simulink model "Question3"  (R2018a)
settings: Solver=VariableStepDiscrete  StartTime=0.0  StopTime=0.5  RelTol=1e-3
libraries: powerlib x17, powerlib_meascontrol x1
settings Model: Creator=bulbu  LastModifiedBy=bulbu

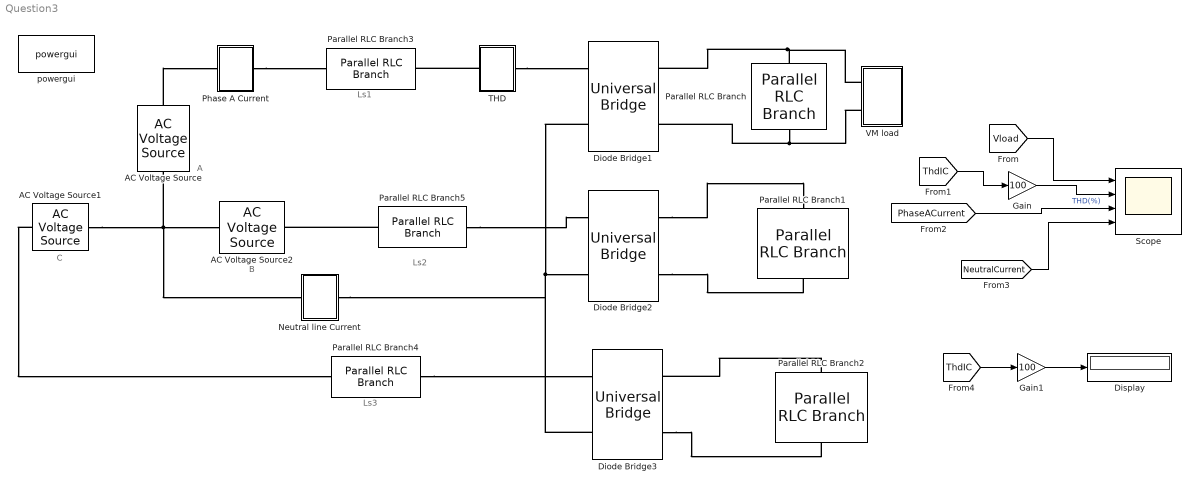
== system Question3 ==
  note: Ls1
  note: C
  note: B
  note: A
  note: Ls2
  note: Ls3
  AC Voltage Source : powerlib/Electrical Sources/AC Voltage Source  Amplitude=326.6  Phase=0  Frequency=50  SampleTime=0  Measurements=None  BusType=swing  Pref=10e3  Qref=0  Qmin=-inf  Qmax=+inf
  AC Voltage Source1 : powerlib/Electrical Sources/AC Voltage Source  Amplitude=326.6  Phase=-120  Frequency=50  SampleTime=0  Measurements=None  BusType=swing  Pref=10e3  Qref=0  Qmin=-inf  Qmax=+inf
  AC Voltage Source2 : powerlib/Electrical Sources/AC Voltage Source  Amplitude=326.6  Phase=120  Frequency=50  SampleTime=0  Measurements=None  BusType=swing  Pref=10e3  Qref=0  Qmin=-inf  Qmax=+inf
  Diode Bridge1 : powerlib/Power Electronics/Universal Bridge  Arms=2  SnubberResistance=1e5  SnubberCapacitance=inf  Device=Diodes  Ron=1e-3  Lon=0  ForwardVoltages="[  0  0  ]"  ForwardVoltage=0  GTOparameters=[ 10e-6 , 20e-6 ]  IGBTparameters=[ 1e-6 , 2e-6 ]  Measurements=None  Measurements_2=None  converterType=Rectifier
  Diode Bridge2 : powerlib/Power Electronics/Universal Bridge  Arms=2  SnubberResistance=1e5  SnubberCapacitance=inf  Device=Diodes  Ron=1e-3  Lon=0  ForwardVoltages="[  0  0  ]"  ForwardVoltage=0  GTOparameters=[ 10e-6 , 20e-6 ]  IGBTparameters=[ 1e-6 , 2e-6 ]  Measurements=None  Measurements_2=None  converterType=Rectifier
  Diode Bridge3 : powerlib/Power Electronics/Universal Bridge  Arms=2  SnubberResistance=1e5  SnubberCapacitance=inf  Device=Diodes  Ron=1e-3  Lon=0  ForwardVoltages="[  0  0  ]"  ForwardVoltage=0  GTOparameters=[ 10e-6 , 20e-6 ]  IGBTparameters=[ 1e-6 , 2e-6 ]  Measurements=None  Measurements_2=None  converterType=Rectifier
  Display : Display
  Gain : Gain  Gain=100
  Gain1 : Gain  Gain=100
  "Neutral line Current " : Subsystem
  Parallel RLC Branch : powerlib/Elements/Parallel RLC Branch  LConnTagsString=a  RConnTagsString=__new0  BranchType=RC  Resistance=200  Inductance=1e-3  SetiL0=off  InitialCurrent=0  Capacitance=470e-6  Setx0=off  InitialVoltage=0  Measurements=None
  Parallel RLC Branch1 : powerlib/Elements/Parallel RLC Branch  LConnTagsString=a  RConnTagsString=__new0  BranchType=RC  Resistance=200  Inductance=1e-3  SetiL0=off  InitialCurrent=0  Capacitance=470e-6  Setx0=off  InitialVoltage=0  Measurements=None
  Parallel RLC Branch2 : powerlib/Elements/Parallel RLC Branch  LConnTagsString=a  RConnTagsString=__new0  BranchType=RC  Resistance=200  Inductance=1e-3  SetiL0=off  InitialCurrent=0  Capacitance=470e-6  Setx0=off  InitialVoltage=0  Measurements=None
  Parallel RLC Branch3 : powerlib/Elements/Parallel RLC Branch  LConnTagsString=a  RConnTagsString=__new0  BranchType=L  Resistance=1  Inductance=600e-6  SetiL0=off  InitialCurrent=0  Capacitance=1e-6  Setx0=off  InitialVoltage=0  Measurements=None
  Parallel RLC Branch4 : powerlib/Elements/Parallel RLC Branch  LConnTagsString=a  RConnTagsString=__new0  BranchType=L  Resistance=1  Inductance=600e-6  SetiL0=off  InitialCurrent=0  Capacitance=1e-6  Setx0=off  InitialVoltage=0  Measurements=None
  Parallel RLC Branch5 : powerlib/Elements/Parallel RLC Branch  LConnTagsString=a  RConnTagsString=__new0  BranchType=L  Resistance=1  Inductance=600e-6  SetiL0=off  InitialCurrent=0  Capacitance=1e-6  Setx0=off  InitialVoltage=0  Measurements=None
  "Phase A Current " : Subsystem
  Scope : Scope  NumInputPorts=4
  THD : Subsystem
  VM load : Subsystem
  powergui : powerlib/powergui  Priority=1  SimulationMode=Discrete  SampleTime=1e-6  frequency=60  Iterations=50  frequencyindice=50  Pbase=100e6  ErrMax=1e-4  UnitsV=kV  UnitsW=MW  buscounter=0  FunctionMessages=off  echomessages=off  EnableUseOfTLC=off  CurrentSourceSwitches=off  DisableSnubberDevices=off  DisableRonSwitches=off  DisableVfSwitches=off  DisplayEquations=off  SolverType=Tustin/Backward Euler (TBE)  Interpol=off  ExternalGateDelay=off  methode=off  Ts=100  x0status=blocks  SPID=on  SwTol=0  HookPort=off  RestoreLinks=warning  ResistiveCurrentMeasurement=off  Frange=[0:2:500]  Ylog=off  Xlog=on  ShowGrid=off  save=off  variable=ZData  structure=0  ZoomFFT=off  StartTime=0.0  cycles=1  DisplayStyle=1  fundamental=60  FreqAxis=off  MaxFrequency=1000  frequencyindicesteady=1  RmsSteady=1  display=off
  wires:
  [Vload] -> Scope/1
  [ThdIC] -> Gain/1
  Gain/1 -> Scope/2  "THD(%)"
  [PhaseACurrent] -> Scope/3
  [NeutralCurrent] -> Scope/4
  [ThdIC] -> Gain1/1
  Gain1/1 -> Display/1
  connections:
  AC Voltage Source1/LConn1 -- "Neutral line Current "/LConn1 -- AC Voltage Source/LConn1 -- AC Voltage Source2/LConn1
  Parallel RLC Branch/LConn1 -- VM load/LConn1 -- Diode Bridge1/RConn1
  Parallel RLC Branch/RConn1 -- VM load/LConn2 -- Diode Bridge1/RConn2
  Diode Bridge2/RConn1 -- Parallel RLC Branch1/LConn1
  Diode Bridge2/RConn2 -- Parallel RLC Branch1/RConn1
  Parallel RLC Branch2/LConn1 -- Diode Bridge3/RConn1
  Diode Bridge3/RConn2 -- Parallel RLC Branch2/RConn1
  AC Voltage Source1/RConn1 -- Parallel RLC Branch4/RConn1
  Parallel RLC Branch4/LConn1 -- Diode Bridge3/LConn1
  Parallel RLC Branch5/LConn1 -- Diode Bridge2/LConn1
  Parallel RLC Branch5/RConn1 -- AC Voltage Source2/RConn1
  THD/LConn1 -- Parallel RLC Branch3/LConn1
  THD/RConn1 -- Diode Bridge1/LConn1
  AC Voltage Source/RConn1 -- "Phase A Current "/LConn1
  "Phase A Current "/RConn1 -- Parallel RLC Branch3/RConn1
  Diode Bridge1/LConn2 -- "Neutral line Current "/RConn1 -- Diode Bridge3/LConn2 -- Diode Bridge2/LConn2

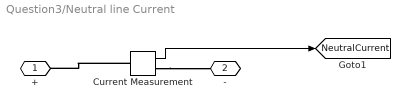
== system Question3/Neutral line Current  ==
  Current Measurement : powerlib/Measurements/Current Measurement  PhasorSimulation=off  OutputType=Complex  PSBequivalent=0
  + : PMIOPort  Side=Left
  - : PMIOPort  Port=2  Side=Right
  tag scope: NeutralCurrent=global
  wires:
  Current Measurement/1 -> [NeutralCurrent]
  connections:
  Current Measurement/RConn1 -- -/RConn1
  Current Measurement/LConn1 -- +/RConn1

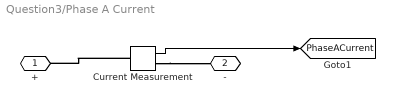
== system Question3/Phase A Current  ==
  Current Measurement : powerlib/Measurements/Current Measurement  PhasorSimulation=off  OutputType=Complex  PSBequivalent=0
  + : PMIOPort  Side=Left
  - : PMIOPort  Port=2  Side=Right
  tag scope: PhaseACurrent=global
  wires:
  Current Measurement/1 -> [PhaseACurrent]
  connections:
  Current Measurement/RConn1 -- -/RConn1
  Current Measurement/LConn1 -- +/RConn1

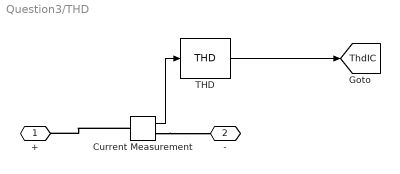
== system Question3/THD ==
  Current Measurement : powerlib/Measurements/Current Measurement  PhasorSimulation=off  OutputType=Complex  PSBequivalent=0
  THD : powerlib_meascontrol/Measurements/THD  Freq=50  Ts=1e-6
  + : PMIOPort  Side=Left
  - : PMIOPort  Port=2  Side=Right
  tag scope: ThdIC=global
  wires:
  THD/1 -> [ThdIC]
  Current Measurement/1 -> THD/1
  connections:
  Current Measurement/RConn1 -- -/RConn1
  Current Measurement/LConn1 -- +/RConn1

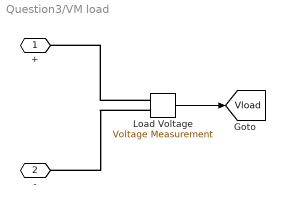
== system Question3/VM load ==
  Load Voltage : powerlib/Measurements/Voltage Measurement  PhasorSimulation=off  OutputType=Complex  PSBequivalent=0
  + : PMIOPort  Side=Left
  - : PMIOPort  Port=2  Side=Left
  tag scope: Vload=global
  wires:
  Load Voltage/1 -> [Vload]
  connections:
  Load Voltage/LConn1 -- +/RConn1
  Load Voltage/LConn2 -- -/RConn1
